simulink model "BMS_AMK_model"  (R2022b)
settings: Solver=FixedStepAuto  StartTime=0.0  StopTime=inf  FixedStep=0.005  RelTol=1e-3
undefined symbols (not defined in the file): canChannel, MI_STATUSES
libraries: canmsglib x19, canlib x14, AMK_comms_plant_lib x1, BMS_plant_lib x1, battery_monitor_lib x1, driver_interface_lib x1, governor_lib x1, motor_interface_lib x1, simp_vd_lib x1
(part 2 of 2)

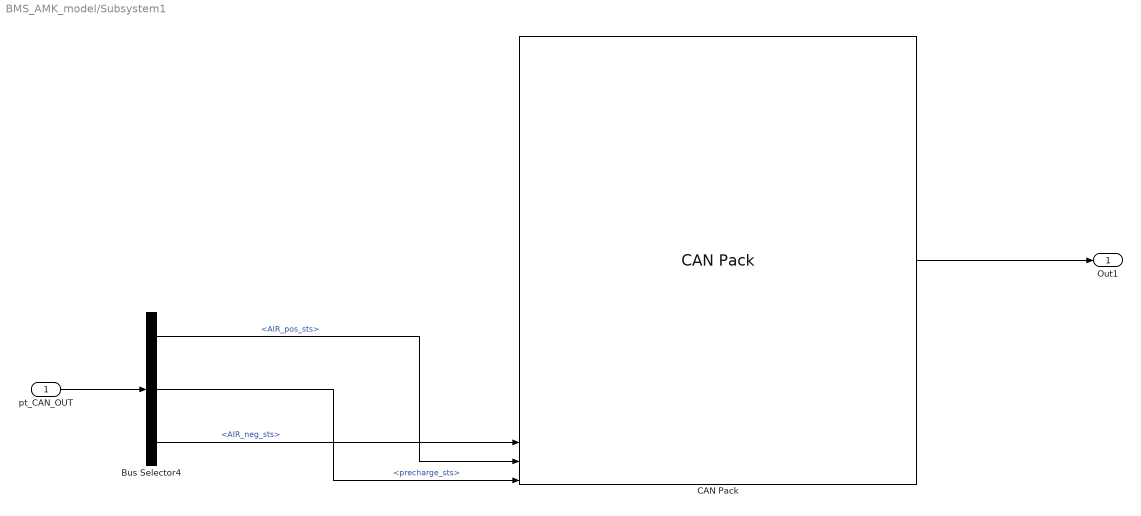
== system BMS_AMK_model/Subsystem1 ==
  pt_CAN_OUT : Inport
  Bus Selector4 : BusSelector  OutputSignals=AIR_pos_sts,precharge_sts,AIR_neg_sts
  CAN Pack : canmsglib/CAN Pack  CANdbFile=C:\Users\LinF\Documents\MACFE\Embedded\CAN_Databases\BMS.dbc  MsgList=MSGID_0X626  MsgName=MSGID_0X626  MsgIDType=Standard (11-bit identifier)  MsgIdentifier=1574  MsgLength=3  Remote=off  ApplyMinMax=off  BusOutput=off  SignalInfo={'Blank','1','1','LE','unsigned','Standard','0','1','0','0','1';'Blank','2','1','LE','unsigned','Standard','0','1','0','0','1';'Blank','3','1','LE','unsigned','Standard','0','1','0','0','1';'Blank','4','1','LE','unsigned','Standard','0','1','0','0','1';'Blank','5','1','LE','unsigned','Standard','0','1','0','0','1';'Blank','6','1','LE','unsigned','Standard','0','1','0','0','1';'Blank','7','1','LE','unsigned','Standard','0','1','0','0','1';'Blank','9','1','LE','unsigned','Standard','0','1','0','0','1';'Blank','10','1','LE','unsigned','Standard','0','1','0','0','1';'Blank','11','1','LE','unsigned','Standard','0','1','0','0','1';'Blank','12','1','LE','unsigned','Standard','0','1','0','0','1';'Blank','13','1','LE','unsigned','Standard','0','1','0','0','1';'Blank','14','1','LE','unsigned','Standard','0','1','0','0','1';'Blank','15','1','LE','unsigned','Standard','0','1','0','0','1';'Blank','17','1','LE','unsigned','Standard','0','1','0','0','1';'Blank','18','1','LE','unsigned','Standard','0','1','0','0','1';'Blank','19','1','LE','unsigned','Standard','0','1','0','0','1';'Blank','20','1','LE','unsigned','Standard','0','1','0','0','1';'Blank','21','1','LE','unsigned','Standard','0','1','0','0','1';'Blank','22','1','LE','unsigned','Standard','0','1','0','0','1';'Blank','23','1','LE','unsigned','Standard','0','1','0','0','1';'MultiPurpose_Output','0','1','LE','unsigned','Standard','0','1','0','0','1';'MultiPurpose_Output_2','8','1','LE','unsigned','Standard','0','1','0','0','1';'MultiPurpose_Output_4','16','1','LE','unsigned','Standard','0','1','0','0','1'}
      settings: LibrarySourceBlock=canlib/CAN Pack  DataFormat=CANdb specified signals
  Out1 : Outport
  wires:
  pt_CAN_OUT/1 -> Bus Selector4/1
  Bus Selector4/1 -> CAN Pack/23  "<AIR_pos_sts>"
  Bus Selector4/2 -> CAN Pack/24  "<precharge_sts>"
  Bus Selector4/3 -> CAN Pack/22  "<AIR_neg_sts>"
  CAN Pack/1 -> Out1/1
